simulink model "COSTEP_Exergy"  (R2024b)
settings: Solver=FixedStepAuto  StartTime=0.0  StopTime=25  FixedStep=1/3600  RelTol=1e-3
model workspace (MAT data in the model file):
  AD : Simulink.Parameter (value not decoded)
  AG : Simulink.Parameter (value not decoded)
  AH : Simulink.Parameter (value not decoded)
  AV : Simulink.Parameter (value not decoded)
  AVP : Simulink.Parameter (value not decoded)
  BCHL : Simulink.Parameter (value not decoded)
  BCHV : Simulink.Parameter (value not decoded)
  BD : Simulink.Parameter (value not decoded)
  BDIST : Simulink.Parameter (value not decoded)
  BG : Simulink.Parameter (value not decoded)
  BH : Simulink.Parameter (value not decoded)
  BVP : Simulink.Parameter (value not decoded)
  CD : Simulink.Parameter (value not decoded)
  CDIST : Simulink.Parameter (value not decoded)
  CG : Simulink.Parameter (value not decoded)
  CH : Simulink.Parameter (value not decoded)
  CVP : Simulink.Parameter (value not decoded)
  DDIST : Simulink.Parameter (value not decoded)
  DIST_CONST : Simulink.Parameter (value not decoded)
  ISV : Simulink.Parameter (value not decoded)
  TLAST : Simulink.Parameter (value not decoded)
  TNEXT : Simulink.Parameter (value not decoded)
  XMW : Simulink.Parameter (value not decoded)
  XNS : Simulink.Parameter (value not decoded)
  XNS2 : Simulink.Parameter (value not decoded)
  XNS3 : Simulink.Parameter (value not decoded)
  XNSADD : Simulink.Parameter (value not decoded)
  XNSE : Simulink.Parameter (value not decoded)
symbols that are objects in the model workspace (value not decoded): AD, AG, AH, AV, AVP, BD, BG, BH, BVP, CD, CG, CH, CVP, XMW, XNS, XNS2, XNS3, XNSE
undefined symbols (not defined in the file or in its folder): magnitude, msgbox, SETPT, XMEAS, XMV
libraries: mylib x403, dspindex x31
(part 7 of 13)

== system COSTEP_Exergy/Separator/Holdup of Components in Separator/Subsystem2 ==
  Bus Creator : BusCreator  Inputs=8
  Bus Selector2 : BusSelector  OutputSignals=signal1.FCM(I;10)
  FCM(1,10) : Gain
  FCM(2,10) : Gain
  FCM(3,10) : Gain
  FCM(4,10) : Gain
  FCM(5,10) : Gain
  FCM(6,10) : Gain
  FCM(7,10) : Gain
  FCM(8,10) : Gain
  Multiport Selector2 : dspindex/Multiport Selector  rowsOrCols=Rows  idxCellArray={ 1,2,3,4,5,6,7,8}  idxErrMode=Clip Index
  FCM(I;10) : Outport  VectorParamsAs1DForOutWhenUnconnected=off
  wires:
  [PropertiesStream10] -> Bus Selector2/1
  FCM(4,10)/1 -> Bus Creator/4  "FCM(4;10)"
  Multiport Selector2/5 -> FCM(5,10)/1
  Multiport Selector2/4 -> FCM(4,10)/1
  FCM(2,10)/1 -> Bus Creator/2  "FCM(2;10)"
  Multiport Selector2/8 -> FCM(8,10)/1
  Multiport Selector2/7 -> FCM(7,10)/1
  FCM(8,10)/1 -> Bus Creator/8  "FCM(8;10)"
  Multiport Selector2/2 -> FCM(2,10)/1
  Multiport Selector2/3 -> FCM(3,10)/1
  Multiport Selector2/1 -> FCM(1,10)/1
  Bus Selector2/1 -> Multiport Selector2/1  "<FCM(I;10)>"
  Multiport Selector2/6 -> FCM(6,10)/1
  FCM(5,10)/1 -> Bus Creator/5  "FCM(5;10)"
  FCM(3,10)/1 -> Bus Creator/3  "FCM(3;10)"
  FCM(1,10)/1 -> Bus Creator/1  "FCM(1;10)"
  FCM(6,10)/1 -> Bus Creator/6  "FCM(6;10)"
  FCM(7,10)/1 -> Bus Creator/7  "FCM(7;10)"
  Bus Creator/1 -> FCM(I;10)/1

== system COSTEP_Exergy/Separator/Holdup of Components in Separator/Subsystem3 ==
  Bus Creator : BusCreator  Inputs=8
  Bus Selector3 : BusSelector  OutputSignals=signal1.FCM(I;11)
  FCM(1,11) : Gain
  FCM(2,11) : Gain
  FCM(3,11) : Gain
  FCM(4,11) : Gain
  FCM(5,11) : Gain
  FCM(6,11) : Gain
  FCM(7,11) : Gain
  FCM(8,11) : Gain
  Multiport Selector3 : dspindex/Multiport Selector  rowsOrCols=Rows  idxCellArray={1,2,3,4,5,6,7,8}  idxErrMode=Clip Index
  FCM(I;11) : Outport  VectorParamsAs1DForOutWhenUnconnected=off
  wires:
  Multiport Selector3/3 -> FCM(3,11)/1
  Multiport Selector3/2 -> FCM(2,11)/1
  Multiport Selector3/5 -> FCM(5,11)/1
  Multiport Selector3/8 -> FCM(8,11)/1
  Bus Selector3/1 -> Multiport Selector3/1  "<FCM(I;11)>"
  Multiport Selector3/7 -> FCM(7,11)/1
  Multiport Selector3/6 -> FCM(6,11)/1
  Multiport Selector3/1 -> FCM(1,11)/1
  Multiport Selector3/4 -> FCM(4,11)/1
  [PropertiesStream11] -> Bus Selector3/1
  FCM(5,11)/1 -> Bus Creator/5  "FCM(5;11)"
  FCM(8,11)/1 -> Bus Creator/8  "FCM(8;11)"
  FCM(7,11)/1 -> Bus Creator/7  "FCM(7;11)"
  FCM(6,11)/1 -> Bus Creator/6  "FCM(6;11)"
  FCM(2,11)/1 -> Bus Creator/2  "FCM(2;11)"
  FCM(3,11)/1 -> Bus Creator/3  "FCM(3;11)"
  FCM(4,11)/1 -> Bus Creator/4  "FCM(4;11)"
  FCM(1,11)/1 -> Bus Creator/1  "FCM(1;11)"
  Bus Creator/1 -> FCM(I;11)/1

== system COSTEP_Exergy/Separator/Holdup of Components in Separator/YP(10) ==
  FCM(1,8) : Inport
  FCM(1,9) : Inport  Port=2
  FCM(1,10) : Inport  Port=3
  FCM(1,11) : Inport  Port=4
  " " : Sum  Inputs=+---
  Bus Selector : BusSelector  OutputSignals=FCM(1;8)
  Bus Selector1 : BusSelector  OutputSignals=FCM(1;9)
  Bus Selector2 : BusSelector  OutputSignals=FCM(1;10)
  Bus Selector3 : BusSelector  OutputSignals=FCM(1;11)
  Constant : Constant  Value=10
  Initial state variable : mylib/Initial state variable
  Integration : mylib/Integration  SystemSampleTime=-1  VariantActivationTime=update diagram  AllowFlexibleInterface=on  Latency=0  AutoFrameSizeCalculation=off
  YY(10) : Outport  VectorParamsAs1DForOutWhenUnconnected=off
  wires:
  Initial state variable/1 -> Integration/2
  FCM(1,10)/1 -> Bus Selector2/1
  FCM(1,9)/1 -> Bus Selector1/1
  FCM(1,8)/1 -> Bus Selector/1
  " "/1 -> Integration/1
  Integration/1 -> YY(10)/1
  FCM(1,11)/1 -> Bus Selector3/1
  Bus Selector/1 -> " "/1  "<FCM(1;8)>"
  Bus Selector1/1 -> " "/2  "<FCM(1;9)>"
  Bus Selector2/1 -> " "/3  "<FCM(1;10)>"
  Bus Selector3/1 -> " "/4  "<FCM(1;11)>"
  Constant/1 -> Initial state variable/1

== system COSTEP_Exergy/Separator/Holdup of Components in Separator/YP(11) ==
  FCM(2,8) : Inport
  FCM(2,9) : Inport  Port=2
  FCM(2,10) : Inport  Port=3
  FCM(2,11) : Inport  Port=4
  " " : Sum  Inputs=+---
  Bus Selector : BusSelector  OutputSignals=FCM(2;8)
  Bus Selector1 : BusSelector  OutputSignals=FCM(2;9)
  Bus Selector2 : BusSelector  OutputSignals=FCM(2;10)
  Bus Selector3 : BusSelector  OutputSignals=FCM(2;11)
  Constant : Constant  Value=11
  Initial state variable : mylib/Initial state variable
  Integration : mylib/Integration  SystemSampleTime=-1  VariantActivationTime=update diagram  AllowFlexibleInterface=on  Latency=0  AutoFrameSizeCalculation=off
  YY(11) : Outport  VectorParamsAs1DForOutWhenUnconnected=off
  wires:
  Integration/1 -> YY(11)/1
  FCM(2,8)/1 -> Bus Selector/1
  FCM(2,9)/1 -> Bus Selector1/1
  FCM(2,10)/1 -> Bus Selector2/1
  FCM(2,11)/1 -> Bus Selector3/1
  Initial state variable/1 -> Integration/2
  " "/1 -> Integration/1
  Bus Selector/1 -> " "/1  "<FCM(2;8)>"
  Bus Selector1/1 -> " "/2  "<FCM(2;9)>"
  Bus Selector2/1 -> " "/3  "<FCM(2;10)>"
  Bus Selector3/1 -> " "/4  "<FCM(2;11)>"
  Constant/1 -> Initial state variable/1

== system COSTEP_Exergy/Separator/Holdup of Components in Separator/YP(12) ==
  FCM(3,8) : Inport
  FCM(3,9) : Inport  Port=2
  FCM(3,10) : Inport  Port=3
  FCM(3,11) : Inport  Port=4
  " " : Sum  Inputs=+---
  Bus Selector : BusSelector  OutputSignals=FCM(3;11)
  Bus Selector1 : BusSelector  OutputSignals=FCM(3;10)
  Bus Selector2 : BusSelector  OutputSignals=FCM(3;9)
  Bus Selector3 : BusSelector  OutputSignals=FCM(3;8)
  Constant : Constant  Value=12
  Initial state variable : mylib/Initial state variable
  Integration : mylib/Integration  SystemSampleTime=-1  VariantActivationTime=update diagram  AllowFlexibleInterface=on  Latency=0  AutoFrameSizeCalculation=off
  YY(12) : Outport  VectorParamsAs1DForOutWhenUnconnected=off
  wires:
  Integration/1 -> YY(12)/1
  FCM(3,8)/1 -> Bus Selector3/1
  FCM(3,9)/1 -> Bus Selector2/1
  FCM(3,10)/1 -> Bus Selector1/1
  FCM(3,11)/1 -> Bus Selector/1
  " "/1 -> Integration/1
  Initial state variable/1 -> Integration/2
  Bus Selector3/1 -> " "/1  "<FCM(3;8)>"
  Bus Selector2/1 -> " "/2  "<FCM(3;9)>"
  Bus Selector1/1 -> " "/3  "<FCM(3;10)>"
  Bus Selector/1 -> " "/4  "<FCM(3;11)>"
  Constant/1 -> Initial state variable/1

== system COSTEP_Exergy/Separator/Holdup of Components in Separator/YP(13) ==
  FCM(4,8) : Inport
  FCM(4,9) : Inport  Port=2
  FCM(4,10) : Inport  Port=3
  FCM(4,11) : Inport  Port=4
  " " : Sum  Inputs=+---
  Bus Selector : BusSelector  OutputSignals=FCM(4;11)
  Bus Selector1 : BusSelector  OutputSignals=FCM(4;10)
  Bus Selector2 : BusSelector  OutputSignals=FCM(4;9)
  Bus Selector3 : BusSelector  OutputSignals=FCM(4;8)
  Constant : Constant  Value=13
  Initial state variable : mylib/Initial state variable
  Integration : mylib/Integration  SystemSampleTime=-1  VariantActivationTime=update diagram  AllowFlexibleInterface=on  Latency=0  AutoFrameSizeCalculation=off
  "YY(13) " : Outport  VectorParamsAs1DForOutWhenUnconnected=off
  wires:
  Integration/1 -> "YY(13) "/1
  FCM(4,8)/1 -> Bus Selector3/1
  FCM(4,9)/1 -> Bus Selector2/1
  FCM(4,10)/1 -> Bus Selector1/1
  FCM(4,11)/1 -> Bus Selector/1
  " "/1 -> Integration/1
  Initial state variable/1 -> Integration/2
  Bus Selector3/1 -> " "/1  "<FCM(4;8)>"
  Bus Selector2/1 -> " "/2  "<FCM(4;9)>"
  Bus Selector1/1 -> " "/3  "<FCM(4;10)>"
  Bus Selector/1 -> " "/4  "<FCM(4;11)>"
  Constant/1 -> Initial state variable/1

== system COSTEP_Exergy/Separator/Holdup of Components in Separator/YP(14) ==
  FCM(5,8) : Inport
  FCM(5,9) : Inport  Port=2
  FCM(5,10) : Inport  Port=3
  FCM(5,11) : Inport  Port=4
  " " : Sum  Inputs=+---
  Bus Selector : BusSelector  OutputSignals=FCM(5;8)
  Bus Selector1 : BusSelector  OutputSignals=FCM(5;9)
  Bus Selector2 : BusSelector  OutputSignals=FCM(5;11)
  Bus Selector3 : BusSelector  OutputSignals=FCM(5;10)
  Constant : Constant  Value=14
  Initial state variable : mylib/Initial state variable
  Integration : mylib/Integration  SystemSampleTime=-1  VariantActivationTime=update diagram  AllowFlexibleInterface=on  Latency=0  AutoFrameSizeCalculation=off
  "YY(14) " : Outport  VectorParamsAs1DForOutWhenUnconnected=off
  wires:
  Integration/1 -> "YY(14) "/1
  FCM(5,8)/1 -> Bus Selector/1
  FCM(5,9)/1 -> Bus Selector1/1
  FCM(5,10)/1 -> Bus Selector3/1
  FCM(5,11)/1 -> Bus Selector2/1
  " "/1 -> Integration/1
  Initial state variable/1 -> Integration/2
  Bus Selector/1 -> " "/1  "<FCM(5;8)>"
  Bus Selector1/1 -> " "/2  "<FCM(5;9)>"
  Bus Selector3/1 -> " "/3  "<FCM(5;10)>"
  Bus Selector2/1 -> " "/4  "<FCM(5;11)>"
  Constant/1 -> Initial state variable/1

== system COSTEP_Exergy/Separator/Holdup of Components in Separator/YP(15) ==
  FCM(6,8) : Inport
  FCM(6,9) : Inport  Port=2
  FCM(6,10) : Inport  Port=3
  FCM(6,11) : Inport  Port=4
  " " : Sum  Inputs=+---
  Bus Selector : BusSelector  OutputSignals=FCM(6;8)
  Bus Selector1 : BusSelector  OutputSignals=FCM(6;11)
  Bus Selector2 : BusSelector  OutputSignals=FCM(6;10)
  Bus Selector3 : BusSelector  OutputSignals=FCM(6;9)
  Constant : Constant  Value=15
  Initial state variable : mylib/Initial state variable
  Integration : mylib/Integration  SystemSampleTime=-1  VariantActivationTime=update diagram  AllowFlexibleInterface=on  Latency=0  AutoFrameSizeCalculation=off
  "YY(15) " : Outport  VectorParamsAs1DForOutWhenUnconnected=off
  wires:
  Integration/1 -> "YY(15) "/1
  FCM(6,8)/1 -> Bus Selector/1
  FCM(6,9)/1 -> Bus Selector3/1
  FCM(6,10)/1 -> Bus Selector2/1
  FCM(6,11)/1 -> Bus Selector1/1
  " "/1 -> Integration/1
  Initial state variable/1 -> Integration/2
  Bus Selector3/1 -> " "/2  "<FCM(6;9)>"
  Bus Selector2/1 -> " "/3  "<FCM(6;10)>"
  Bus Selector1/1 -> " "/4  "<FCM(6;11)>"
  Bus Selector/1 -> " "/1  "<FCM(6;8)>"
  Constant/1 -> Initial state variable/1

== system COSTEP_Exergy/Separator/Holdup of Components in Separator/YP(16) ==
  FCM(7,8) : Inport
  FCM(7,9) : Inport  Port=2
  FCM(7,10) : Inport  Port=3
  FCM(7,11) : Inport  Port=4
  " " : Sum  Inputs=+---
  Bus Selector : BusSelector  OutputSignals=FCM(7;11)
  Bus Selector1 : BusSelector  OutputSignals=FCM(7;10)
  Bus Selector2 : BusSelector  OutputSignals=FCM(7;9)
  Bus Selector3 : BusSelector  OutputSignals=FCM(7;8)
  Constant : Constant  Value=16
  Initial state variable : mylib/Initial state variable
  Integration : mylib/Integration  SystemSampleTime=-1  VariantActivationTime=update diagram  AllowFlexibleInterface=on  Latency=0  AutoFrameSizeCalculation=off
  "YY(16) " : Outport  VectorParamsAs1DForOutWhenUnconnected=off
  wires:
  Integration/1 -> "YY(16) "/1
  FCM(7,8)/1 -> Bus Selector3/1
  FCM(7,9)/1 -> Bus Selector2/1
  FCM(7,10)/1 -> Bus Selector1/1
  FCM(7,11)/1 -> Bus Selector/1
  " "/1 -> Integration/1
  Initial state variable/1 -> Integration/2
  Bus Selector3/1 -> " "/1  "<FCM(7;8)>"
  Bus Selector2/1 -> " "/2  "<FCM(7;9)>"
  Bus Selector1/1 -> " "/3  "<FCM(7;10)>"
  Bus Selector/1 -> " "/4  "<FCM(7;11)>"
  Constant/1 -> Initial state variable/1

== system COSTEP_Exergy/Separator/Holdup of Components in Separator/YP(17) ==
  FCM(8,8) : Inport
  FCM(8,9) : Inport  Port=2
  FCM(8,10) : Inport  Port=3
  FCM(8,11) : Inport  Port=4
  " " : Sum  Inputs=+---
  Bus Selector : BusSelector  OutputSignals=FCM(8;11)
  Bus Selector1 : BusSelector  OutputSignals=FCM(8;10)
  Bus Selector2 : BusSelector  OutputSignals=FCM(8;9)
  Bus Selector3 : BusSelector  OutputSignals=FCM(8;8)
  Constant : Constant  Value=17
  Initial state variable : mylib/Initial state variable
  Integration : mylib/Integration  SystemSampleTime=-1  VariantActivationTime=update diagram  AllowFlexibleInterface=on  Latency=0  AutoFrameSizeCalculation=off
  "YY(17) " : Outport  VectorParamsAs1DForOutWhenUnconnected=off
  wires:
  Integration/1 -> "YY(17) "/1
  FCM(8,8)/1 -> Bus Selector3/1
  FCM(8,9)/1 -> Bus Selector2/1
  FCM(8,10)/1 -> Bus Selector1/1
  " "/1 -> Integration/1
  Initial state variable/1 -> Integration/2
  FCM(8,11)/1 -> Bus Selector/1
  Bus Selector3/1 -> " "/1  "<FCM(8;8)>"
  Bus Selector2/1 -> " "/2  "<FCM(8;9)>"
  Bus Selector1/1 -> " "/3  "<FCM(8;10)>"
  Bus Selector/1 -> " "/4  "<FCM(8;11)>"
  Constant/1 -> Initial state variable/1

== system COSTEP_Exergy/Separator/Pressure of Separator/Subsystem ==
  TCS : Inport
  VVS : Inport  Port=2
  UCVS : Inport  Port=3
  Bus Selector : BusSelector  OutputSignals=UCVS(1),UCVS(2),UCVS(3)
  PPS(1) Partial pressure of Component A mmHg : Product  Inputs=***/
  PPS(2) Partial pressure of Component B mmHg : Product  Inputs=***/
  PPS(3) Partial pressure of Component C mmHg : Product  Inputs=***/
  RG Universal Gas Constant ft³·mmHg/K·lb-mol : Constant  Value=998.9
  TKS Temperature in Separator K : Sum
  To Convert °C to K : Constant  Value=273.15
  PPS(1) : Outport  VectorParamsAs1DForOutWhenUnconnected=off
  PPS(2) : Outport  Port=2  VectorParamsAs1DForOutWhenUnconnected=off
  PPS(3) : Outport  Port=3  VectorParamsAs1DForOutWhenUnconnected=off
  wires:
  Bus Selector/3 -> PPS(3) Partial pressure of Component C mmHg/1  "<UCVS(3)>"
  RG Universal Gas Constant ft³·mmHg/K·lb-mol/1 -> PPS(3) Partial pressure of Component C mmHg/2, PPS(1) Partial pressure of Component A mmHg/2, PPS(2) Partial pressure of Component B mmHg/2
  UCVS/1 -> Bus Selector/1
  Bus Selector/1 -> PPS(1) Partial pressure of Component A mmHg/1  "<UCVS(1)>"
  Bus Selector/2 -> PPS(2) Partial pressure of Component B mmHg/1  "<UCVS(2)>"
  VVS/1 -> PPS(3) Partial pressure of Component C mmHg/4, PPS(2) Partial pressure of Component B mmHg/4, PPS(1) Partial pressure of Component A mmHg/4
  PPS(3) Partial pressure of Component C mmHg/1 -> PPS(3)/1
  To Convert °C to K/1 -> TKS Temperature in Separator K/2
  PPS(1) Partial pressure of Component A mmHg/1 -> PPS(1)/1
  TKS Temperature in Separator K/1 -> PPS(3) Partial pressure of Component C mmHg/3, PPS(2) Partial pressure of Component B mmHg/3, PPS(1) Partial pressure of Component A mmHg/3
  PPS(2) Partial pressure of Component B mmHg/1 -> PPS(2)/1
  TCS/1 -> TKS Temperature in Separator K/1

== system COSTEP_Exergy/Separator/Pressure of Separator/VPR Vapour Pressure mmHg ==
  TCS : Inport
  AVP(I) Antoine Coefficient A ln(mmHg) : Constant  Value=AVP
  Add : Sum
  Add1 : Sum
  BVP(I) Antoine Coefficient B ln(mmHg)·°C : Constant  Value=BVP
  CVP(I) Antoine Coefficient C °C : Constant  Value=CVP
  Divide : Product  Inputs=*/
  Math Function : Math  SignedPower=on
  VPR : Outport  VectorParamsAs1DForOutWhenUnconnected=off
  wires:
  BVP(I) Antoine Coefficient B ln(mmHg)·°C/1 -> Divide/1
  CVP(I) Antoine Coefficient C °C/1 -> Add/1
  AVP(I) Antoine Coefficient A ln(mmHg)/1 -> Add1/1
  Add/1 -> Divide/2
  Divide/1 -> Add1/2
  Add1/1 -> Math Function/1
  Math Function/1 -> VPR/1
  TCS/1 -> Add/2

== system COSTEP_Exergy/Separator/Stream 10/HST(10) Molar Enthalpy of Stream 10 MBtu//lb-mol ==
  ITY : Inport
  T : Inport  Port=2
  XST(I,I) : Inport  Port=3
  "Enthalpy of Stream " : mylib/Enthalpy of Stream   SystemSampleTime=-1  VariantActivationTime=update diagram  AllowFlexibleInterface=on  Latency=0  AutoFrameSizeCalculation=off
  "H " : Outport  VectorParamsAs1DForOutWhenUnconnected=off
  wires:
  ITY/1 -> "Enthalpy of Stream "/1
  T/1 -> "Enthalpy of Stream "/2
  XST(I,I)/1 -> "Enthalpy of Stream "/3
  "Enthalpy of Stream "/1 -> "H "/1

== system COSTEP_Exergy/Separator/Stream 10/Subsystem ==
  VPOS(6) : Inport  PortDimensions=1
  Abs : Abs  SaturateOnIntegerOverflow=off
  Constant : Constant  Value=0.0
  Constant1 : Constant  Value=0.151169
  Constant2 : Constant  Value=760
  DLP : Sum  Inputs=+-
  DLP Pressure drop between separator and environment : Merge
  FLMS : Product  Inputs=3
  If : If  IfExpression=u1 < 0
  If Action Subsystem : Subsystem  TreatAsAtomicUnit=on
  If Action Subsystem1 : Subsystem  TreatAsAtomicUnit=on
  Sqrt : Sqrt
  Out1 : Outport  VectorParamsAs1DForOutWhenUnconnected=off
  wires:
  Constant2/1 -> DLP/2
  Constant1/1 -> FLMS/2
  Abs/1 -> Sqrt/1
  DLP Pressure drop between separator and environment/1 -> Abs/1
  [PTS] -> DLP/1
  If Action Subsystem/1(Out1) -> DLP Pressure drop between separator and environment/1
  Constant/1 -> If Action Subsystem/1(In1)
  Sqrt/1 -> FLMS/3
  If Action Subsystem1/1(Out1) -> DLP Pressure drop between separator and environment/2
  If/2 -> If Action Subsystem1/Action
  DLP/1 -> If Action Subsystem1/1(In1), If/1
  VPOS(6)/1 -> FLMS/1
  If/1 -> If Action Subsystem/Action
  FLMS/1 -> Out1/1

== system COSTEP_Exergy/Separator/Stream 10/XMWS(10) Molecular weight of Stream 10 lb//lb-mol ==
  XST(I,10) : Inport
  Constant : Constant  Value=XMW
  Product : Product
  Sum of Elements : Sum  Inputs=+
  XMWS(10) : Outport  VectorParamsAs1DForOutWhenUnconnected=off
  wires:
  Sum of Elements/1 -> XMWS(10)/1
  Product/1 -> Sum of Elements/1
  XST(I,10)/1 -> Product/1
  Constant/1 -> Product/2

== system COSTEP_Exergy/Separator/Stream 11/HST(10) Molar Enthalpy of Stream 10 MBtu//lb-mol ==
  ITY : Inport
  T : Inport  Port=2
  XST(I,I) : Inport  Port=3
  "Enthalpy of Stream " : mylib/Enthalpy of Stream   SystemSampleTime=-1  VariantActivationTime=update diagram  AllowFlexibleInterface=on  Latency=0  AutoFrameSizeCalculation=off
  "H " : Outport  VectorParamsAs1DForOutWhenUnconnected=off
  wires:
  ITY/1 -> "Enthalpy of Stream "/1
  T/1 -> "Enthalpy of Stream "/2
  XST(I,I)/1 -> "Enthalpy of Stream "/3
  "Enthalpy of Stream "/1 -> "H "/1

== system COSTEP_Exergy/Separator/Stream 11/PTSL Pressure of Liquid From Separator mmHg ==
  XLS : Inport
  TCS : Inport  Port=2
  Bus Creator1 : BusCreator  Inputs=8
  Demux : Demux  Outputs=8
  PPR(I) : Product
  PTSL Total Pressure of liquid from Separator mmHg : Sum  Inputs=+
  VPR Vapour Pressure mmHg : Subsystem
  PTSL : Outport  PortDimensions=1  VectorParamsAs1DForOutWhenUnconnected=off
  wires:
  Demux/1 -> Bus Creator1/1  "PPR(1)"
  Demux/2 -> Bus Creator1/2  "PPR(2)"
  Demux/7 -> Bus Creator1/7  "PPR(7)"
  TCS/1 -> VPR Vapour Pressure mmHg/1(TCR)
  Demux/8 -> Bus Creator1/8  "PPR(8)"
  PPR(I)/1 -> Demux/1
  VPR Vapour Pressure mmHg/1(VPR) -> PPR(I)/2
  PTSL Total Pressure of liquid from Separator mmHg/1 -> PTSL/1
  XLS/1 -> PPR(I)/1
  Bus Creator1/1 -> PTSL Total Pressure of liquid from Separator mmHg/1
  Demux/6 -> Bus Creator1/6  "PPR(6)"
  Demux/4 -> Bus Creator1/4  "PPR(4)"
  Demux/5 -> Bus Creator1/5  "PPR(5)"
  Demux/3 -> Bus Creator1/3  "PPR(3)"

== system COSTEP_Exergy/Separator/Stream 9/HST(9) Molar Enthalpy of Stream 9 MBtu//lb-mol ==
  ITY : Inport
  T : Inport  Port=2
  XST(I,I) : Inport  Port=3
  "Enthalpy of Stream " : mylib/Enthalpy of Stream   SystemSampleTime=-1  VariantActivationTime=update diagram  AllowFlexibleInterface=on  Latency=0  AutoFrameSizeCalculation=off
  "H " : Outport  PortDimensions=1  VectorParamsAs1DForOutWhenUnconnected=off
  wires:
  ITY/1 -> "Enthalpy of Stream "/1
  T/1 -> "Enthalpy of Stream "/2
  XST(I,I)/1 -> "Enthalpy of Stream "/3
  "Enthalpy of Stream "/1 -> "H "/1

== system COSTEP_Exergy/Separator/Stream 9/Subsystem ==
  VPOS(5) : Inport
  Abs : Abs  SaturateOnIntegerOverflow=off
  Constant1 : Constant  Value=53.349
  Constant2 : Constant  Value=1E-3
  FLMS : Product  Inputs=3
  "FLMS  " : Merge
  If Action Subsystem2 : Subsystem  TreatAsAtomicUnit=on
  If Action Subsystem3 : Subsystem  TreatAsAtomicUnit=on
  If1 : If  IfExpression=u1 < 1E-3
  Pressure drop : Subsystem
  Sqrt : Sqrt
  Subtract : Sum  Inputs=+-
  "FLMS " : Outport  VectorParamsAs1DForOutWhenUnconnected=off
  wires:
  FLMS/1 -> Subtract/2
  If1/1 -> If Action Subsystem2/Action
  [FLMS] -> Subtract/1
  Subtract/1 -> If Action Subsystem3/1(In1), If1/1
  If Action Subsystem3/1(Out1) -> "FLMS  "/2
  Abs/1 -> Sqrt/1
  Constant1/1 -> FLMS/2
  Sqrt/1 -> FLMS/3
  If1/2 -> If Action Subsystem3/Action
  Constant2/1 -> If Action Subsystem2/1(In1)
  VPOS(5)/1 -> FLMS/1
  If Action Subsystem2/1(Out1) -> "FLMS  "/1
  "FLMS  "/1 -> "FLMS "/1
  Pressure drop/1("DLP ") -> Abs/1

== system COSTEP_Exergy/Separator/Stream 9/XMWS(9) Molecular weight of Stream 9 lb//lb-mol ==
  XST(I,9) : Inport
  Product : Product
  Sum of Elements : Sum  Inputs=+
  "XMW(I) Molecular weight of components lb/lb-mol " : Constant  Value=[2;25.4;28;32;46;48;62;76]
  XMWS(9) : Outport  VectorParamsAs1DForOutWhenUnconnected=off
  wires:
  Sum of Elements/1 -> XMWS(9)/1
  Product/1 -> Sum of Elements/1
  XST(I,9)/1 -> Product/1
  "XMW(I) Molecular weight of components lb/lb-mol "/1 -> Product/2

== system COSTEP_Exergy/Separator/Volume of Separator/DLS Molar Density of Liquids in Reactor lb-mol//ft³     ==
  XLS : Inport
  TCS : Inport  Port=2
  "DLS Molar Density of Liquids in Separator lb-mol/ft³ " : Subsystem
  "DLS " : Outport  VectorParamsAs1DForOutWhenUnconnected=off
  wires:
  "DLS Molar Density of Liquids in Separator lb-mol/ft³ "/1("R ") -> "DLS "/1
  TCS/1 -> "DLS Molar Density of Liquids in Separator lb-mol/ft³ "/2(T)
  XLS/1 -> "DLS Molar Density of Liquids in Separator lb-mol/ft³ "/1(X)

== system COSTEP_Exergy/Stream Measurements/Subsystem6/A and C feed stream ==
  Stream 4 : Inport
  Bus Creator : BusCreator  Inputs=4
  Bus Selector : BusSelector  OutputSignals=XMNSE(7),XMNSE(8)
  Bus Selector1 : BusSelector  OutputSignals=TST(4),XST(I;4)
  Bus Selector2 : BusSelector  OutputSignals=Stream 4
  Bus Selector3 : BusSelector  OutputSignals=signal1.XMEAS(4)
  Composition measurement mol% : Subsystem
  Constant : Constant  Value=1000
  Flow measurement in kg/h : Subsystem
  Pressure measurement in kPa : Subsystem
  Temperature measurement in C : Subsystem
  tag scope: SM4=global
  wires:
  Bus Selector1/1 -> Temperature measurement in C/1(T in celsius)  "<TST(4)>"
  Temperature measurement in C/1(SMEAST(4)) -> Bus Creator/1  "SMEAST(4)"
  [XMNSE] -> Bus Selector/1
  Bus Selector/1 -> Temperature measurement in C/2(XMNSE)  "<XMNSE(7)>"
  Bus Selector/2 -> Pressure measurement in kPa/2(XMNSE)  "<XMNSE(8)>"
  Stream 4/1 -> Bus Selector1/1
  Bus Selector1/2 -> Flow measurement in kg/h/2(XST), Composition measurement mol%/1(XST)  "<XST(I;4)>"
  Constant/1 -> Pressure measurement in kPa/1("P in mm Hg ")
  Pressure measurement in kPa/1(SMEASP(4)) -> Bus Creator/2  "SMEASP(4)"
  Flow measurement in kg/h/1("SMEASF(4) ") -> Bus Creator/3  "SMEASF(4)"
  Composition measurement mol%/1(SMEASX(4)) -> Bus Creator/4  "SMEASX(4)"
  Bus Creator/1 -> [SM4]
  [XMNSE2] -> Bus Selector2/1
  Bus Selector2/1 -> Composition measurement mol%/2(XMNSE)  "<Stream 4>"
  [XMEAS] -> Bus Selector3/1
  Bus Selector3/1 -> Flow measurement in kg/h/1(XMEAS in kscmh)  "<XMEAS(4)>"

== system COSTEP_Exergy/Stream Measurements/Subsystem6/A feed stream ==
  Stream 3 : Inport
  Bus Creator : BusCreator  Inputs=4
  Bus Selector : BusSelector  OutputSignals=XMNSE(5),XMNSE(6)
  Bus Selector1 : BusSelector  OutputSignals=TST(3),XST(I;3)
  Bus Selector2 : BusSelector  OutputSignals=Stream 3
  Bus Selector3 : BusSelector  OutputSignals=signal1.XMEAS(1)
  Composition measurement mol% : Subsystem
  Constant : Constant  Value=1000
  Flow measurement in kg/h : Subsystem
  Pressure measurement in kPa : Subsystem
  Temperature measurement in C : Subsystem
  tag scope: SM1=global
  wires:
  Bus Selector1/1 -> Temperature measurement in C/1(T in celsius)  "<TST(3)>"
  Temperature measurement in C/1(SMEAST(1)) -> Bus Creator/1  "SMEAST(1)"
  [XMNSE] -> Bus Selector/1
  Bus Selector/1 -> Temperature measurement in C/2(XMNSE)  "<XMNSE(5)>"
  Bus Selector/2 -> Pressure measurement in kPa/2(XMNSE)  "<XMNSE(6)>"
  Stream 3/1 -> Bus Selector1/1
  Bus Selector1/2 -> Flow measurement in kg/h/2(XST), Composition measurement mol%/1(XST)  "<XST(I;3)>"
  Constant/1 -> Pressure measurement in kPa/1("P in mm Hg ")
  Pressure measurement in kPa/1(SMEASP(1)) -> Bus Creator/2  "SMEASP(1)"
  Flow measurement in kg/h/1("SMEASF(1) ") -> Bus Creator/3  "SMEASF(1)"
  Composition measurement mol%/1(SMEASX(1)) -> Bus Creator/4  "SMEASX(1)"
  Bus Creator/1 -> [SM1]
  [XMNSE2] -> Bus Selector2/1
  Bus Selector2/1 -> Composition measurement mol%/2(XMNSE)  "<Stream 3>"
  [XMEAS] -> Bus Selector3/1
  Bus Selector3/1 -> Flow measurement in kg/h/1(XMEAS in kscmh)  "<XMEAS(1)>"

== system COSTEP_Exergy/Stream Measurements/Subsystem6/CCIn ==
  Bus Creator : BusCreator  Inputs=3
  Bus Selector : BusSelector  OutputSignals=XMNSE(20),XMNSE(21),XMNSE(22)
  Flow measurement in kg/h : Subsystem
  Pressure measurement in kPa : Subsystem
  Temperature measurement in C : Subsystem
  tag scope: SM17=global
  wires:
  [TCWS] -> Pressure measurement in kPa/2(TC), Temperature measurement in C/1(T in celsius)
  Bus Creator/1 -> [SM17]
  [FWS] -> Flow measurement in kg/h/2(F in gpm)
  [XMNSE] -> Bus Selector/1
  Bus Selector/1 -> Temperature measurement in C/2(XMNSE)  "<XMNSE(20)>"
  Bus Selector/2 -> Pressure measurement in kPa/1(XMNSE)  "<XMNSE(21)>"
  Bus Selector/3 -> Flow measurement in kg/h/1(XMNSE)  "<XMNSE(22)>"
  Temperature measurement in C/1(SMEAST) -> Bus Creator/1
  Pressure measurement in kPa/1(SMEASP) -> Bus Creator/2
  Flow measurement in kg/h/1("SMEASF ") -> Bus Creator/3

== system COSTEP_Exergy/Stream Measurements/Subsystem6/CCOut ==
  Bus Creator : BusCreator  Inputs=2
  Bus Selector : BusSelector  OutputSignals=XMNSE(23),XMNSE(24)
  Pressure measurement in kPa : Subsystem
  Temperature measurement in C : Subsystem
  tag scope: SM13=global
  wires:
  [TWS] -> Pressure measurement in kPa/2(TC), Temperature measurement in C/1(T in celsius)
  Bus Creator/1 -> [SM13]
  [XMNSE] -> Bus Selector/1
  Bus Selector/1 -> Temperature measurement in C/2(XMNSE)  "<XMNSE(23)>"
  Bus Selector/2 -> Pressure measurement in kPa/1(XMNSE)  "<XMNSE(24)>"
  Temperature measurement in C/1(SMEAST) -> Bus Creator/1
  Pressure measurement in kPa/1(SMEASP) -> Bus Creator/2

== system COSTEP_Exergy/Stream Measurements/Subsystem6/Condenser product stream ==
  Stream 8 : Inport
  Bus Creator : BusCreator  Inputs=4
  Bus Selector : BusSelector  OutputSignals=XMNSE(12)
  Bus Selector1 : BusSelector  OutputSignals=signal1.XST(I;8),signal1.FTM(8),signal1.HST(8),signal1.Phase
  Bus Selector2 : BusSelector  OutputSignals=Stream 8
  Bus Selector3 : BusSelector  OutputSignals=signal2.XMEAS(7)
  Composition measurement mol% : Subsystem
  Flow measurement in kg/h : Subsystem
  Pressure measurement in kPa : Subsystem
  Subsystem : Subsystem
  Temperature measurement in C : Subsystem
  tag scope: SM14=global
  wires:
  Temperature measurement in C/1(SMEAST) -> Bus Creator/1
  [XMNSE] -> Bus Selector/1
  Stream 8/1 -> Bus Selector1/1
  Bus Selector1/1 -> Subsystem/2(XST), Composition measurement mol%/1(XST), Flow measurement in kg/h/1(XST)  "<XST(I;8)>"
  Pressure measurement in kPa/1(SMEASP) -> Bus Creator/2
  Flow measurement in kg/h/1("SMEASF ") -> Bus Creator/3
  Composition measurement mol%/1(SMEASX) -> Bus Creator/4
  Bus Creator/1 -> [SM14]
  [XMNSE2] -> Bus Selector2/1
  Bus Selector2/1 -> Composition measurement mol%/2(XMNSE)  "<Stream 8>"
  [XMEAS] -> Bus Selector3/1
  Bus Selector3/1 -> Pressure measurement in kPa/1(XMEAS in kPa gauge)  "<XMEAS(7)>"
  Bus Selector1/2 -> Flow measurement in kg/h/3(F in lb-mol/h)  "<FTM(8)>"
  Bus Selector/1 -> Flow measurement in kg/h/2(XMNSE)  "<XMNSE(12)>"
  Subsystem/1(TST(8a)) -> Temperature measurement in C/1(XMEAS in celsius)
  Bus Selector1/3 -> Subsystem/1(HST(8))  "<HST(8)>"
  Bus Selector1/4 -> Subsystem/3(ITY)  "<Phase>"

== system COSTEP_Exergy/Stream Measurements/Subsystem6/D feed stream ==
  Stream 1 : Inport
  Bus Creator : BusCreator  Inputs=4
  Bus Selector : BusSelector  OutputSignals=XMNSE(1),XMNSE(2)
  Bus Selector1 : BusSelector  OutputSignals=TST(1),XST(I;1)
  Bus Selector2 : BusSelector  OutputSignals=Stream 1
  Bus Selector3 : BusSelector  OutputSignals=signal1.XMEAS(2)
  Composition measurement mol% : Subsystem
  Constant : Constant  Value=1000
  Flow measurement in kg/h : Subsystem
  Pressure measurement in kPa : Subsystem
  Temperature measurement in C : Subsystem
  tag scope: SM2=global
  wires:
  Bus Selector1/1 -> Temperature measurement in C/1(T in celsius)  "<TST(1)>"
  Temperature measurement in C/1(SMEAST(2)) -> Bus Creator/1  "SMEAST(2)"
  [XMNSE] -> Bus Selector/1
  Bus Selector/1 -> Temperature measurement in C/2(XMNSE)  "<XMNSE(1)>"
  Bus Selector/2 -> Pressure measurement in kPa/2(XMNSE)  "<XMNSE(2)>"
  Stream 1/1 -> Bus Selector1/1
  Bus Selector1/2 -> Composition measurement mol%/1(XST)  "<XST(I;1)>"
  Constant/1 -> Pressure measurement in kPa/1("P in mm Hg ")
  Pressure measurement in kPa/1(SMEASP(2)) -> Bus Creator/2  "SMEASP(2)"
  Flow measurement in kg/h/1("SMEASF(2) ") -> Bus Creator/3  "SMEASF(2)"
  Composition measurement mol%/1(SMEASX(2)) -> Bus Creator/4  "SMEASX(2)"
  Bus Creator/1 -> [SM2]
  [XMNSE2] -> Bus Selector2/1
  Bus Selector2/1 -> Composition measurement mol%/2(XMNSE)  "<Stream 1>"
  [XMEAS] -> Bus Selector3/1
  Bus Selector3/1 -> Flow measurement in kg/h/1(XMEAS in kg/h)  "<XMEAS(2)>"

== system COSTEP_Exergy/Stream Measurements/Subsystem6/E feed stream ==
  Stream 2 : Inport
  Bus Creator : BusCreator  Inputs=4
  Bus Selector : BusSelector  OutputSignals=XMNSE(3),XMNSE(4)
  Bus Selector1 : BusSelector  OutputSignals=TST(2),XST(I;2)
  Bus Selector2 : BusSelector  OutputSignals=Stream 2
  Bus Selector3 : BusSelector  OutputSignals=signal1.XMEAS(3)
  Composition measurement mol% : Subsystem
  Constant : Constant  Value=1000
  Flow measurement in kg/h : Subsystem
  Pressure measurement in kPa : Subsystem
  Temperature measurement in C : Subsystem
  tag scope: SM3=global
  wires:
  Bus Selector1/1 -> Temperature measurement in C/1(T in celsius)  "<TST(2)>"
  Temperature measurement in C/1(SMEAST(3)) -> Bus Creator/1  "SMEAST(3)"
  [XMNSE] -> Bus Selector/1
  Bus Selector/1 -> Temperature measurement in C/2(XMNSE)  "<XMNSE(3)>"
  Bus Selector/2 -> Pressure measurement in kPa/2(XMNSE)  "<XMNSE(4)>"
  Stream 2/1 -> Bus Selector1/1
  Bus Selector1/2 -> Composition measurement mol%/1(XST)  "<XST(I;2)>"
  Constant/1 -> Pressure measurement in kPa/1("P in mm Hg ")
  Pressure measurement in kPa/1(SMEASP(3)) -> Bus Creator/2  "SMEASP(3)"
  Flow measurement in kg/h/1("SMEASF(3) ") -> Bus Creator/3  "SMEASF(3)"
  Composition measurement mol%/1(SMEASX(3)) -> Bus Creator/4  "SMEASX(3)"
  Bus Creator/1 -> [SM3]
  [XMNSE2] -> Bus Selector2/1
  Bus Selector2/1 -> Composition measurement mol%/2(XMNSE)  "<Stream 2>"
  [XMEAS] -> Bus Selector3/1
  Bus Selector3/1 -> Flow measurement in kg/h/1(XMEAS in kg/h)  "<XMEAS(3)>"

== system COSTEP_Exergy/Stream Measurements/Subsystem6/Product stream ==
  Stream 13 : Inport
  Bus Creator : BusCreator  Inputs=4
  Bus Selector : BusSelector  OutputSignals=XMNSE(14)
  Bus Selector1 : BusSelector  OutputSignals=PTC,XST(I;13)
  Bus Selector2 : BusSelector  OutputSignals=Stream 13
  Bus Selector3 : BusSelector  OutputSignals=signal4.XMEAS(18),signal4.XMEAS(17)
  Bus Selector4 : BusSelector  OutputSignals=Stream 13
  Composition measurement mol% : Subsystem
  Flow measurement in kg/h : Subsystem
  Pressure measurement in kPa : Subsystem
  Temperature measurement in C : Subsystem
  tag scope: SM11=global
  wires:
  Temperature measurement in C/1(SMEAST) -> Bus Creator/1
  [XMNSE] -> Bus Selector/1
  Stream 13/1 -> Bus Selector1/1
  Pressure measurement in kPa/1(SMEASP) -> Bus Creator/2
  Flow measurement in kg/h/1("SMEASF ") -> Bus Creator/3  "SMEASF"
  Composition measurement mol%/1(SMEASX) -> Bus Creator/4
  Bus Creator/1 -> [SM11]
  [XMNSE2] -> Bus Selector2/1
  Bus Selector2/1 -> Composition measurement mol%/2(XMNSE2)  "<Stream 13>"
  [XMEAS] -> Bus Selector3/1
  Bus Selector/1 -> Pressure measurement in kPa/2(XMNSE)  "<XMNSE(14)>"
  Bus Selector1/1 -> Pressure measurement in kPa/1("P in mm Hg ")  "<PTC>"
  Bus Selector3/1 -> Temperature measurement in C/1(XMEAS in celsius)  "<XMEAS(18)>"
  Bus Selector3/2 -> Flow measurement in kg/h/1(XMEAS in m^3/h)  "<XMEAS(17)>"
  Bus Selector1/2 -> Composition measurement mol%/1(XST), Flow measurement in kg/h/2(XST)  "<XST(I;13)>"
  [XMNSE3] -> Bus Selector4/1
  Bus Selector4/1 -> Composition measurement mol%/3(XMNSE3)  "<Stream 13>"

== system COSTEP_Exergy/Stream Measurements/Subsystem6/Purge stream ==
  Stream 10 : Inport
  Bus Creator : BusCreator  Inputs=4
  Bus Selector : BusSelector  OutputSignals=XMNSE(2)
  Bus Selector1 : BusSelector  OutputSignals=signal1.XST(I;10)
  Bus Selector3 : BusSelector  OutputSignals=signal3.XMEAS(11),signal3.XMEAS(10),signal9
  Composition measurement mol% : Subsystem
  Flow measurement in kg/h : Subsystem
  Pressure measurement in kPa : Subsystem
  Temperature measurement in C : Subsystem
  tag scope: SM9=global
  wires:
  Temperature measurement in C/1(SMEAST(9)) -> Bus Creator/1  "SMEAST(9)"
  Stream 10/1 -> Bus Selector1/1
  Bus Selector1/1 -> Flow measurement in kg/h/2(XST)  "<XST(I;10)>"
  Pressure measurement in kPa/1(SMEASP(9)) -> Bus Creator/2  "SMEASP(9)"
  Flow measurement in kg/h/1("SMEASF(9) ") -> Bus Creator/3  "SMEASF(9)"
  Composition measurement mol%/1(SMEASX(9)) -> Bus Creator/4  "SMEASX(9)"
  Bus Creator/1 -> [SM9]
  [XMEAS] -> Bus Selector3/1
  Bus Selector3/1 -> Temperature measurement in C/1(XMEAS in celsius)  "<XMEAS(11)>"
  Bus Selector3/2 -> Flow measurement in kg/h/1(XMEAS in kscmh)  "<XMEAS(10)>"
  Bus Selector3/3 -> Composition measurement mol%/1(XMEAS)  "<signal9>"
  [XMNSE] -> Bus Selector/1
  Bus Selector/1 -> Pressure measurement in kPa/1(XMNSE)  "<XMNSE(2)>"

== system COSTEP_Exergy/Stream Measurements/Subsystem6/RCIn ==
  Bus Creator : BusCreator  Inputs=3
  Bus Selector : BusSelector  OutputSignals=XMNSE(15),XMNSE(16),XMNSE(17)
  Flow measurement in kg/h : Subsystem
  Pressure measurement in kPa : Subsystem
  Temperature measurement in C : Subsystem
  tag scope: SM16=global
  wires:
  [TCWR] -> Pressure measurement in kPa/2(TC), Temperature measurement in C/1(T in celsius)
  [FWR] -> Flow measurement in kg/h/2(F in gpm)
  [XMNSE] -> Bus Selector/1
  Bus Selector/1 -> Temperature measurement in C/2(XMNSE)  "<XMNSE(15)>"
  Bus Selector/2 -> Pressure measurement in kPa/1(XMNSE)  "<XMNSE(16)>"
  Bus Selector/3 -> Flow measurement in kg/h/1(XMNSE)  "<XMNSE(17)>"
  Temperature measurement in C/1(SMEAST) -> Bus Creator/1
  Pressure measurement in kPa/1(SMEASP) -> Bus Creator/2
  Flow measurement in kg/h/1("SMEASF ") -> Bus Creator/3
  Bus Creator/1 -> [SM16]

== system COSTEP_Exergy/Stream Measurements/Subsystem6/RCOut ==
  Bus Creator : BusCreator  Inputs=2
  Bus Selector : BusSelector  OutputSignals=XMNSE(18),XMNSE(19)
  Pressure measurement in kPa : Subsystem
  Temperature measurement in C : Subsystem
  tag scope: SM12=global
  wires:
  [TWR] -> Pressure measurement in kPa/2(TC), Temperature measurement in C/1(T in celsius)
  Bus Creator/1 -> [SM12]
  [XMNSE] -> Bus Selector/1
  Bus Selector/1 -> Temperature measurement in C/2(XMNSE)  "<XMNSE(18)>"
  Bus Selector/2 -> Pressure measurement in kPa/1(XMNSE)  "<XMNSE(19)>"
  Temperature measurement in C/1(SMEAST) -> Bus Creator/1
  Pressure measurement in kPa/1(SMEASP) -> Bus Creator/2

== system COSTEP_Exergy/Stream Measurements/Subsystem6/Reactor feed stream ==
  Stream 6 : Inport
  Bus Creator : BusCreator  Inputs=4
  Bus Selector : BusSelector  OutputSignals=XMNSE(11)
  Bus Selector1 : BusSelector  OutputSignals=signal1.TST(6) = TST(7),signal1.XST(I;6) = XST(I;7)
  Bus Selector2 : BusSelector  OutputSignals=Stream 6
  Bus Selector3 : BusSelector  OutputSignals=signal4.XMEAS(16),signal2.XMEAS(6),signal8
  Composition measurement mol% : Subsystem
  Flow measurement in kg/h : Subsystem
  Pressure measurement in kPa : Subsystem
  Temperature measurement in C : Subsystem
  tag scope: SM6=global
  wires:
  Bus Selector1/1 -> Temperature measurement in C/1(T in celsius)  "<TST(6) = TST(7)>"
  Temperature measurement in C/1(SMEAST) -> Bus Creator/1  "SMEAST(6)"
  [XMNSE] -> Bus Selector/1
  Bus Selector/1 -> Temperature measurement in C/2(XMNSE)  "<XMNSE(11)>"
  Stream 6/1 -> Bus Selector1/1
  Bus Selector1/2 -> Flow measurement in kg/h/2(XST), Composition measurement mol%/1(XST)  "<XST(I;6) = XST(I;7)>"
  [XMEAS] -> Bus Selector3/1
  Pressure measurement in kPa/1(SMEASP) -> Bus Creator/2  "SMEASP(6)"
  Flow measurement in kg/h/1("SMEASF ") -> Bus Creator/3  "SMEASF(6)"
  Composition measurement mol%/1(SMEASX(6)) -> Bus Creator/4  "SMEASX(6)"
  Bus Creator/1 -> [SM6]
  [XMNSE2] -> Bus Selector2/1
  Bus Selector2/1 -> Composition measurement mol%/2(XMNSE)  "<Stream 6>"
  Bus Selector3/1 -> Pressure measurement in kPa/1(XMEAS in kPa gauge)  "<XMEAS(16)>"
  Bus Selector3/2 -> Flow measurement in kg/h/1(XMEAS in kscmh)  "<XMEAS(6)>"
  Bus Selector3/3 -> Composition measurement mol%/3(XMEAS)  "<signal8>"

== system COSTEP_Exergy/Stream Measurements/Subsystem6/Reactor product stream ==
  Stream 8 : Inport
  Bus Creator : BusCreator  Inputs=4
  Bus Selector : BusSelector  OutputSignals=XMNSE(12)
  Bus Selector1 : BusSelector  OutputSignals=signal1.XST(I;8),signal1.FTM(8)
  Bus Selector2 : BusSelector  OutputSignals=Stream 8
  Bus Selector3 : BusSelector  OutputSignals=signal2.XMEAS(9),signal2.XMEAS(7)
  Composition measurement mol% : Subsystem
  Flow measurement in kg/h : Subsystem
  Pressure measurement in kPa : Subsystem
  Temperature measurement in C : Subsystem
  tag scope: SM7=global
  wires:
  Temperature measurement in C/1(SMEAST(7)) -> Bus Creator/1  "SMEAST(7)"
  [XMNSE] -> Bus Selector/1
  Stream 8/1 -> Bus Selector1/1
  Bus Selector1/1 -> Composition measurement mol%/1(XST), Flow measurement in kg/h/1(XST)  "<XST(I;8)>"
  Pressure measurement in kPa/1(SMEASP(7)) -> Bus Creator/2  "SMEASP(7)"
  Flow measurement in kg/h/1("SMEASF(7) ") -> Bus Creator/3  "SMEASF(7)"
  Composition measurement mol%/1(SMEASX(7)) -> Bus Creator/4  "SMEASX(7)"
  Bus Creator/1 -> [SM7]
  [XMNSE2] -> Bus Selector2/1
  Bus Selector2/1 -> Composition measurement mol%/2(XMNSE)  "<Stream 8>"
  [XMEAS] -> Bus Selector3/1
  Bus Selector3/1 -> Temperature measurement in C/1(XMEAS in celsius)  "<XMEAS(9)>"
  Bus Selector3/2 -> Pressure measurement in kPa/1(XMEAS in kPa gauge)  "<XMEAS(7)>"
  Bus Selector1/2 -> Flow measurement in kg/h/3(F in lb-mol/h)  "<FTM(8)>"
  Bus Selector/1 -> Flow measurement in kg/h/2(XMNSE)  "<XMNSE(12)>"

== system COSTEP_Exergy/Stream Measurements/Subsystem6/Separator product stream ==
  Stream 9 : Inport
  Bus Creator : BusCreator  Inputs=4
  Bus Selector1 : BusSelector  OutputSignals=signal2.XST(I;9)
  Bus Selector2 : BusSelector  OutputSignals=Stream 9
  Bus Selector3 : BusSelector  OutputSignals=signal3.XMEAS(11),signal3.XMEAS(13),signal1.XMEAS(5),signal3.XMEAS(10)
  Composition measurement mol% : Subsystem
  Flow measurement in kg/h : Subsystem
  Pressure measurement in kPa : Subsystem
  Temperature measurement in C : Subsystem
  tag scope: SMNA=global
  wires:
  Temperature measurement in C/1(SMEAST) -> Bus Creator/1  "SMEAST"
  Stream 9/1 -> Bus Selector1/1
  Bus Selector1/1 -> Flow measurement in kg/h/2(XST), Composition measurement mol%/1(XST)  "<XST(I;9)>"
  Pressure measurement in kPa/1(SMEASP) -> Bus Creator/2
  Flow measurement in kg/h/1("SMEASF ") -> Bus Creator/3  "SMEASF"
  Composition measurement mol%/1(SMEASX) -> Bus Creator/4
  Bus Creator/1 -> [SMNA]
  [XMNSE2] -> Bus Selector2/1
  Bus Selector2/1 -> Composition measurement mol%/2(XMNSE)  "<Stream 9>"
  [XMEAS] -> Bus Selector3/1
  Bus Selector3/1 -> Temperature measurement in C/1(XMEAS in celsius)  "<XMEAS(11)>"
  Bus Selector3/2 -> Pressure measurement in kPa/1(XMEAS in kPa gauge)  "<XMEAS(13)>"
  Bus Selector3/3 -> Flow measurement in kg/h/1(XMEAS in kscmh)  "<XMEAS(5)>"
  Bus Selector3/4 -> Flow measurement in kg/h/3(XMEAS in kscmh1)  "<XMEAS(10)>"

== system COSTEP_Exergy/Stream Measurements/Subsystem6/Separator recycle stream (after compressor) ==
  Stream 9 : Inport
  Bus Creator : BusCreator  Inputs=4
  Bus Selector1 : BusSelector  OutputSignals=signal2.XST(I;9),signal2.HST(9),signal2.Phase
  Bus Selector2 : BusSelector  OutputSignals=Stream 9
  Bus Selector3 : BusSelector  OutputSignals=signal4.XMEAS(16),signal1.XMEAS(5)
  Composition measurement mol% : Subsystem
  Flow measurement in kg/h : Subsystem
  Pressure measurement in kPa : Subsystem
  Temperature measurement in C : Subsystem
  tag scope: SM8=global
  wires:
  Temperature measurement in C/1(SMEAST(8)) -> Bus Creator/1  "SMEAST(8)"
  Stream 9/1 -> Bus Selector1/1
  Bus Selector1/1 -> Temperature measurement in C/2(XST), Flow measurement in kg/h/2(XST), Composition measurement mol%/1(XST)  "<XST(I;9)>"
  Pressure measurement in kPa/1(SMEASP(8)) -> Bus Creator/2  "SMEASP(8)"
  Flow measurement in kg/h/1("SMEASF(8) ") -> Bus Creator/3  "SMEASF(8)"
  Composition measurement mol%/1(SMEASX(8)) -> Bus Creator/4  "SMEASX(8)"
  Bus Creator/1 -> [SM8]
  [XMNSE2] -> Bus Selector2/1
  Bus Selector2/1 -> Composition measurement mol%/2(XMNSE)  "<Stream 9>"
  [XMEAS] -> Bus Selector3/1
  Bus Selector3/1 -> Pressure measurement in kPa/1(XMEAS in kPa gauge)  "<XMEAS(16)>"
  Bus Selector3/2 -> Flow measurement in kg/h/1(XMEAS in kscmh)  "<XMEAS(5)>"
  Bus Selector1/2 -> Temperature measurement in C/1(HST(9))  "<HST(9)>"
  Bus Selector1/3 -> Temperature measurement in C/3(ITY)  "<Phase>"

== system COSTEP_Exergy/Stream Measurements/Subsystem6/Separator recycle stream (before compressor) ==
  Stream 9 : Inport
  Bus Creator : BusCreator  Inputs=4
  Bus Selector1 : BusSelector  OutputSignals=signal2.XST(I;9)
  Bus Selector2 : BusSelector  OutputSignals=Stream 9
  Bus Selector3 : BusSelector  OutputSignals=signal3.XMEAS(11),signal3.XMEAS(13),signal1.XMEAS(5)
  Composition measurement mol% : Subsystem
  Flow measurement in kg/h : Subsystem
  Pressure measurement in kPa : Subsystem
  Temperature measurement in C : Subsystem
  tag scope: SM15=global
  wires:
  Temperature measurement in C/1(SMEAST) -> Bus Creator/1  "SMEAST"
  Stream 9/1 -> Bus Selector1/1
  Bus Selector1/1 -> Flow measurement in kg/h/2(XST), Composition measurement mol%/1(XST)  "<XST(I;9)>"
  Pressure measurement in kPa/1(SMEASP) -> Bus Creator/2
  Flow measurement in kg/h/1("SMEASF ") -> Bus Creator/3  "SMEASF"
  Composition measurement mol%/1(SMEASX) -> Bus Creator/4
  Bus Creator/1 -> [SM15]
  [XMNSE2] -> Bus Selector2/1
  Bus Selector2/1 -> Composition measurement mol%/2(XMNSE)  "<Stream 9>"
  [XMEAS] -> Bus Selector3/1
  Bus Selector3/1 -> Temperature measurement in C/1(XMEAS in celsius)  "<XMEAS(11)>"
  Bus Selector3/2 -> Pressure measurement in kPa/1(XMEAS in kPa gauge)  "<XMEAS(13)>"
  Bus Selector3/3 -> Flow measurement in kg/h/1(XMEAS in kscmh)  "<XMEAS(5)>"

== system COSTEP_Exergy/Stream Measurements/Subsystem6/Separator underflow stream ==
  Stream 11 : Inport
  Bus Creator : BusCreator  Inputs=4
  Bus Selector1 : BusSelector  OutputSignals=signal1.PTSL,signal1.XST(I;11)
  Bus Selector2 : BusSelector  OutputSignals=Stream 11
  Bus Selector3 : BusSelector  OutputSignals=signal3.XMEAS(11),signal3.XMEAS(14)
  Bus Selector4 : BusSelector  OutputSignals=XMNSE(13)
  Composition measurement mol% : Subsystem
  Flow measurement in kg/h : Subsystem
  Pressure measurement in kPa : Subsystem
  Temperature measurement in C : Subsystem
  tag scope: SM10=global
  wires:
  Temperature measurement in C/1(SMEAST) -> Bus Creator/1
  [XMNSE] -> Bus Selector4/1
  Stream 11/1 -> Bus Selector1/1
  Pressure measurement in kPa/1(SMEASP) -> Bus Creator/2
  Flow measurement in kg/h/1("SMEASF ") -> Bus Creator/3  "SMEASF"
  Composition measurement mol%/1(SMEASX) -> Bus Creator/4
  Bus Creator/1 -> [SM10]
  [XMNSE3] -> Bus Selector2/1
  Bus Selector2/1 -> Composition measurement mol%/2(XMNSE)  "<Stream 11>"
  [XMEAS] -> Bus Selector3/1
  Bus Selector4/1 -> Pressure measurement in kPa/2(XMNSE)  "<XMNSE(13)>"
  Bus Selector1/1 -> Pressure measurement in kPa/1("P in mm Hg ")  "<PTSL>"
  Bus Selector1/2 -> Flow measurement in kg/h/2(XST), Composition measurement mol%/1(XST)  "<XST(I;11)>"
  Bus Selector3/1 -> Temperature measurement in C/1(XMEAS in celsius)  "<XMEAS(11)>"
  Bus Selector3/2 -> Flow measurement in kg/h/1(XMEAS in m^3/h)  "<XMEAS(14)>"

== system COSTEP_Exergy/Stream Measurements/Subsystem6/Stripper recycle stream ==
  Stream 5 : Inport
  Bus Creator : BusCreator  Inputs=4
  Bus Selector : BusSelector  OutputSignals=XMNSE(9),XMNSE(10)
  Bus Selector1 : BusSelector  OutputSignals=TST(5),XST(I;5),FTM(5)
  Bus Selector2 : BusSelector  OutputSignals=Stream 5
  Bus Selector3 : BusSelector  OutputSignals=signal4.XMEAS(16)
  Composition measurement mol% : Subsystem
  Flow measurement in kg/h : Subsystem
  Pressure measurement in kPa : Subsystem
  Temperature measurement in C : Subsystem
  tag scope: SM5=global
  wires:
  Bus Selector1/1 -> Temperature measurement in C/1(T in celsius)  "<TST(5)>"
  Temperature measurement in C/1(SMEAST(5)) -> Bus Creator/1  "SMEAST(5)"
  [XMNSE] -> Bus Selector/1
  Bus Selector/1 -> Temperature measurement in C/2(XMNSE)  "<XMNSE(9)>"
  Stream 5/1 -> Bus Selector1/1
  Bus Selector1/2 -> Composition measurement mol%/1(XST), Flow measurement in kg/h/1(XST)  "<XST(I;5)>"
  [XMEAS] -> Bus Selector3/1
  Pressure measurement in kPa/1(SMEASP(5)) -> Bus Creator/2  "SMEASP(5)"
  Flow measurement in kg/h/1("SMEASF(5) ") -> Bus Creator/3  "SMEASF(5)"
  Composition measurement mol%/1(SMEASX(5)) -> Bus Creator/4  "SMEASX(5)"
  Bus Creator/1 -> [SM5]
  [XMNSE2] -> Bus Selector2/1
  Bus Selector2/1 -> Composition measurement mol%/2(XMNSE)  "<Stream 5>"
  Bus Selector3/1 -> Pressure measurement in kPa/1(XMEAS in kPa gauge)  "<XMEAS(16)>"
  Bus Selector1/3 -> Flow measurement in kg/h/3(F in lb-mol/h)  "<FTM(5)>"
  Bus Selector/2 -> Flow measurement in kg/h/2(XMNSE)  "<XMNSE(10)>"

== system COSTEP_Exergy/Stripper/Heat transfer of stripper/If Action Subsystem ==
  In1 : Inport
  Action Port : ActionPort  ActionPortLabel=if(u1 < 100)
  Out1 : Outport  VectorParamsAs1DForOutWhenUnconnected=off
  wires:
  In1/1 -> Out1/1

== system COSTEP_Exergy/Stripper/Heat transfer of stripper/If Action Subsystem1 ==
  In1 : Inport
  Action Port : ActionPort  ActionPortLabel=else
  Out1 : Outport  VectorParamsAs1DForOutWhenUnconnected=off
  wires:
  In1/1 -> Out1/1
